simulink model "bms"  (R2021a)
settings: Solver=VariableStepAuto  StartTime=0.0  StopTime=10.0  RelTol=1e-3
undefined symbols (not defined in the file or in its folder): BMSBatteryPackInput, BMSContactorModuleCmd, BusSOCEstimation
settings Model: Creator=miche  LastModifiedBy=miche

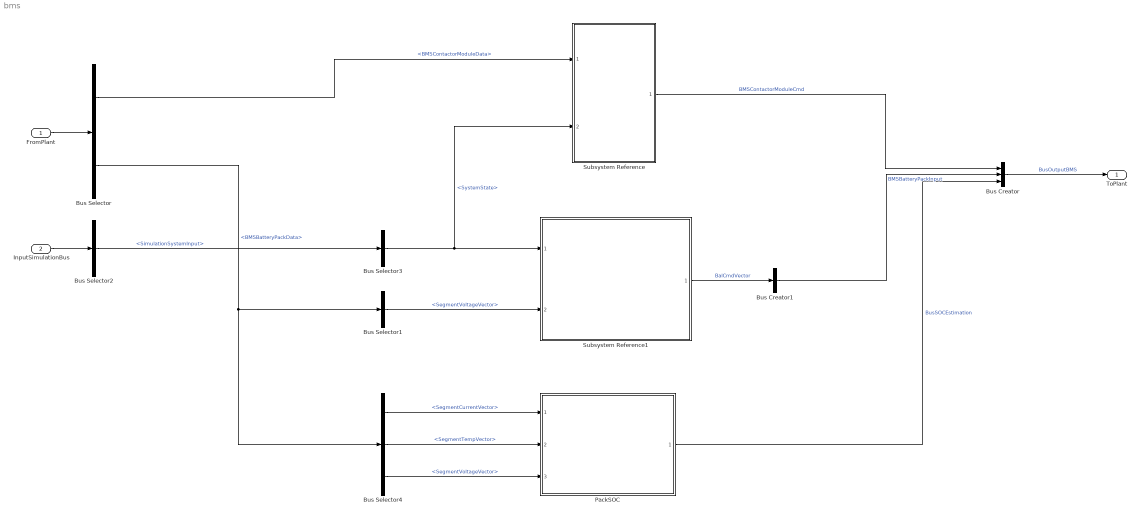
== system bms ==
  FromPlant : Inport  OutDataTypeStr=Bus: BusInputBMS
  InputSimulationBus : Inport  Port=2  OutDataTypeStr=Bus: BusSimulationInput
  Bus Creator : BusCreator  Inputs=BMSContactorModuleCmd,BMSBatteryPackInput,BusSOCEstimation  OutDataTypeStr=Bus: BusOutputBMS
  Bus Creator1 : BusCreator  Inputs=BalCmdVector  OutDataTypeStr=Bus: BMSBatteryPackInput
  Bus Selector : BusSelector  OutputSignals=BMSContactorModuleData,BMSBatteryPackData
  Bus Selector1 : BusSelector  OutputSignals=SegmentVoltageVector
  Bus Selector2 : BusSelector  OutputSignals=SimulationSystemInput
  Bus Selector3 : BusSelector  OutputSignals=SystemState
  Bus Selector4 : BusSelector  OutputSignals=SegmentCurrentVector,SegmentTempVector,SegmentVoltageVector
  PackSOC : Subsystem  ReferencedSubsystem=PackSOC
  Subsystem Reference : Subsystem  ReferencedSubsystem=contactor_logic
  Subsystem Reference1 : Subsystem  ReferencedSubsystem=passive_balancing_logic
  ToPlant : Outport  OutDataTypeStr=Bus: BusOutputBMS
  wires:
  Subsystem Reference/1 -> Bus Creator/1  "BMSContactorModuleCmd"
  Subsystem Reference1/1 -> Bus Creator1/1  "BalCmdVector"
  Bus Creator1/1 -> Bus Creator/2  "BMSBatteryPackInput"
  Bus Creator/1 -> ToPlant/1  "BusOutputBMS"
  FromPlant/1 -> Bus Selector/1
  Bus Selector/1 -> Subsystem Reference/1  "<BMSContactorModuleData>"
  Bus Selector/2 -> Bus Selector4/1, Bus Selector1/1  "<BMSBatteryPackData>"
  Bus Selector1/1 -> Subsystem Reference1/2  "<SegmentVoltageVector>"
  InputSimulationBus/1 -> Bus Selector2/1
  Bus Selector2/1 -> Bus Selector3/1  "<SimulationSystemInput>"
  Bus Selector3/1 -> Subsystem Reference/2, Subsystem Reference1/1  "<SystemState>"
  Bus Selector4/1 -> PackSOC/1  "<SegmentCurrentVector>"
  Bus Selector4/3 -> PackSOC/3  "<SegmentVoltageVector>"
  PackSOC/1 -> Bus Creator/3  "BusSOCEstimation"
  Bus Selector4/2 -> PackSOC/2  "<SegmentTempVector>"
